simulink model "Parallel2"  (Simulink 5.0)
settings: Solver=ode45  StartTime=0.0  StopTime=10.0  RelTol=1e-3
settings Model: Creator=scaife  LastModifiedBy=scaife  ExtModeAutoUpdateStatusClock=off

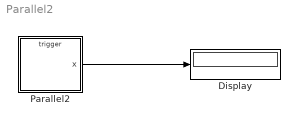
== system Parallel2 ==
  Display : Display
  Parallel2 : Stateflow chart
  wires:
  Parallel2/1(x) -> Display/1

== stateflow chart Parallel2 ==
  state TOP/ en:x+=1000000; ex:x-=1000000;
    state N1/ [parallel]
      en:x+=10000;
      ex:x-=10000;
      state A/
        en: x+=10;
      state B/
        en: x-=10;
      (default) -> A
      A -> B : S1
          | {x+=1;}
      B -> A : R1
          | {x-=1;}
    state N2/ [parallel]
      en:x+=100000;
      ex:x-=100000;
      state C/
        en: x+=1000;
      state D/
        en: x-=1000;
      (default) -> C
      C -> D : S2
          | {x+=100;}
      D -> C : R2
          | {x-=100;}
  (default) -> TOP/ en:x+=1000000; ex:x-=1000000;
  data: x output double
  events: S1 input EITHER_EDGE_EVENT; R1 input EITHER_EDGE_EVENT; S2 input EITHER_EDGE_EVENT; R2 input EITHER_EDGE_EVENT
